simulink model "MotorModelo"  (R2025a)
settings: Solver=VariableStepAuto  StartTime=0.0  StopTime=20  RelTol=1e-3
values from neighbouring files (symbols this model uses):
  B = p0(2)    [DC_Motor.m]    (also in Parametros_Motor.m = 0.0024079912)
  J = p0(1)    [DC_Motor.m]    (also in Parametros_Motor.m = 5.66646261e-05)
  Ka = p0(3)    [DC_Motor.m]    (also in Parametros_Motor.m = 0.2303506651)
  Km = p0(4)    [DC_Motor.m]    (also in Parametros_Motor.m = 0.2303506651)
  L = p0(6)    [DC_Motor.m]    (also in Parametros_Motor.m = 0.0124)
  R = p0(5)    [DC_Motor.m]    (also in Parametros_Motor.m = 23.4)
settings Model: Creator=Sergio  LastModifiedBy=mario
settings SolverCC: AlgebraicLoopSolver=TrustRegion
settings DataIOCC: ReturnWorkspaceOutputs=off
settings DebuggingCC: UnconnectedInputMsg=warning  UnconnectedOutputMsg=warning  UnconnectedLineMsg=warning  ArithmeticOperatorsInVariantConditions=warning
settings ModelReferenceCC: EnableRefExpFcnMdlSchedulingChecks=on
settings SFSimCC: SimUseLocalCustomCode=off  CustomCodeUndefinedFunction=UseInterfaceOnly
settings RTWCC: RTWUseLocalCustomCode=off  GPUComputeCapability=3.5  DLArmComputeVersion=19.05

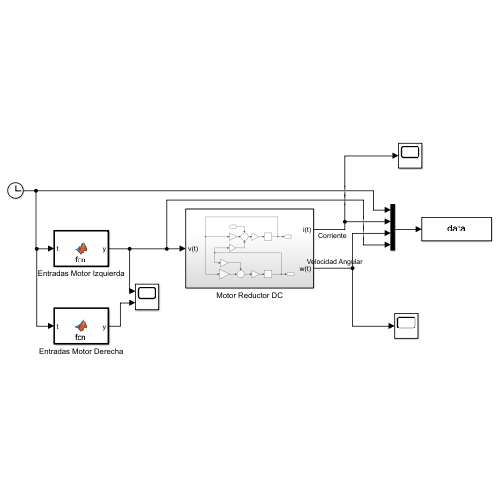
[thumbnail: Simulink's stored preview of the top-level diagram]
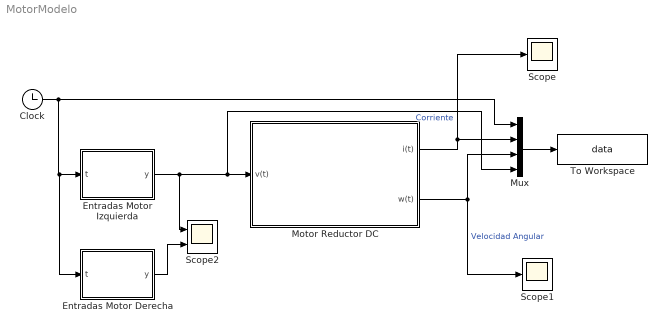
== system MotorModelo ==
  Clock : Clock
  Entradas Motor Derecha : MATLAB Function  TreatAsAtomicUnit=on
  Entradas Motor Izquierda : MATLAB Function  TreatAsAtomicUnit=on
  Motor Reductor DC : Subsystem
  Mux : Mux
  Scope : Scope
      settings: ActiveDisplayYMinimum=-0.27416688110980636  ActiveDisplayYMaximum=0.51193008866824385
  Scope1 : Scope
      settings: ActiveDisplayYMinimum=-2.1494752472241085  ActiveDisplayYMaximum=19.32959654165586
  Scope2 : Scope  NumInputPorts=2
      settings: DataLoggingVariableName=ScopeData2
  To Workspace : ToWorkspace  VariableName=data  SampleTime=0.05
  wires:
  Motor Reductor DC/2(w(t)) -> Scope1/1, Mux/3  "Velocidad Angular"
  Mux/1 -> To Workspace/1
  Clock/1 -> Mux/1, Entradas Motor Derecha/1(t), Entradas Motor Izquierda/1(t)
  Motor Reductor DC/1(i(t)) -> Scope/1, Mux/2  "Corriente"
  Entradas Motor Derecha/1(y) -> Scope2/2
  Entradas Motor Izquierda/1(y) -> Mux/4, Motor Reductor DC/1(v(t)), Scope2/1

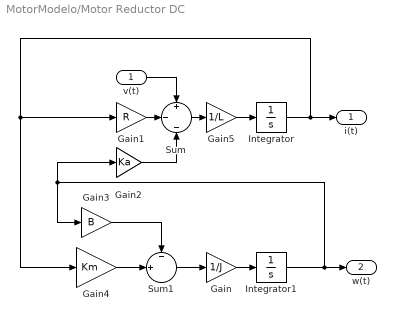
== system MotorModelo/Motor Reductor DC ==
  v(t) : Inport
  Gain : Gain  Gain=1/J
  Gain1 : Gain  Gain=R
  Gain2 : Gain  Gain=Ka
  Gain3 : Gain  Gain=B
  Gain4 : Gain  Gain=Km
  Gain5 : Gain  Gain=1/L
  Integrator : Integrator
  Integrator1 : Integrator
  Sum : Sum  Inputs=+|-|-
  Sum1 : Sum  Inputs=-|+||
  i(t) : Outport  VectorParamsAs1DForOutWhenUnconnected=off
  w(t) : Outport  Port=2  VectorParamsAs1DForOutWhenUnconnected=off
  wires:
  v(t)/1 -> Sum/1
  Gain1/1 -> Sum/2
  Integrator/1 -> i(t)/1, Gain1/1, Gain4/1
  Gain2/1 -> Sum/3
  Integrator1/1 -> Gain3/1, Gain2/1, w(t)/1
  Sum1/1 -> Gain/1
  Gain4/1 -> Sum1/2
  Gain3/1 -> Sum1/1
  Gain5/1 -> Integrator/1
  Sum/1 -> Gain5/1
  Gain/1 -> Integrator1/1

== matlab function MotorModelo/Entradas Motor Izquierda ==
  data: t input; y output
function y = fcn(t)
    if t < 2
        y = 0;
    elseif t < 4
        y = 10.8;
    elseif t < 6
        y = 0;
    elseif t < 8
        y = 8.5;
    elseif t < 10
        y = 0;
    elseif t < 12
        y = 6.3;
    elseif t < 14
        y = 0;
    elseif t < 16
        y = 4.2;
    elseif t < 18
        y = 0;
    else
        y =  2.2;
    end

== matlab function MotorModelo/Entradas Motor Derecha ==
  data: t input; y output
function y = fcn(t)
    if t < 2
        y = 0;
    elseif t < 4
        y = 10.8;
    elseif t < 6
        y = 0;
    elseif t < 8
        y = 8.3;
    elseif t < 10
        y = 0;
    elseif t < 12
        y = 6.1;
    elseif t < 14
        y = 0;
    elseif t < 16
        y = 4.1;
    elseif t < 18
        y = 0;
    else
        y =  2.1;
    end
